simulink model "lista1_7b"  (R2020b)
settings: Solver=VariableStepAuto  StartTime=0.0  StopTime=20  RelTol=1e-3
settings Model: Creator=lucas  LastModifiedBy=lucas

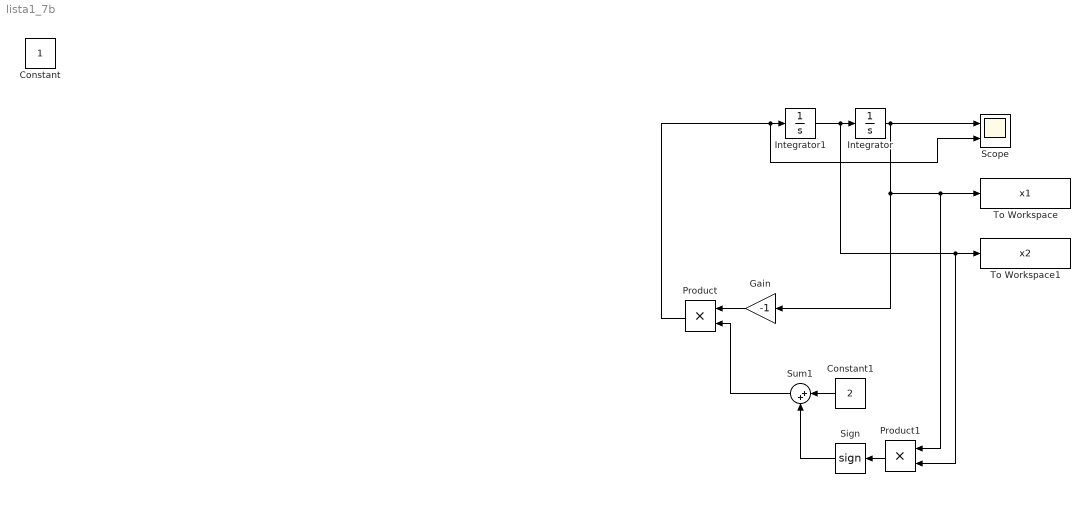
== system lista1_7b ==
  Constant1 : Constant  Value=2
  Gain : Gain  Gain=-1
  Integrator : Integrator  InitialCondition=1
  Integrator1 : Integrator
  Product : Product
  Product1 : Product
  Scope : Scope  NumInputPorts=2
  Sign : Signum
  Sum1 : Sum  Inputs=|++
  To Workspace : ToWorkspace  VariableName=x1  SaveFormat=Timeseries  SampleTime=-1
  To Workspace1 : ToWorkspace  VariableName=x2  SaveFormat=Timeseries  SampleTime=-1
  Constant : Constant  IOType=siggen
  wires:
  Integrator1/1 -> Product1/2, To Workspace1/1, Integrator/1
  Integrator/1 -> Product1/1, To Workspace/1, Gain/1, Scope/1
  Gain/1 -> Product/1
  Constant1/1 -> Sum1/1
  Sign/1 -> Sum1/2
  Product1/1 -> Sign/1
  Sum1/1 -> Product/2
  Product/1 -> Scope/2, Integrator1/1
